simulink model "Discrete_PID_Rotate_to_Angle"  (R2020a)
settings: Solver=VariableStepAuto  StartTime=0.0  StopTime=10.0  RelTol=1e-3
libraries: simulink x2
settings Model: Creator=tieub  LastModifiedBy=tieub

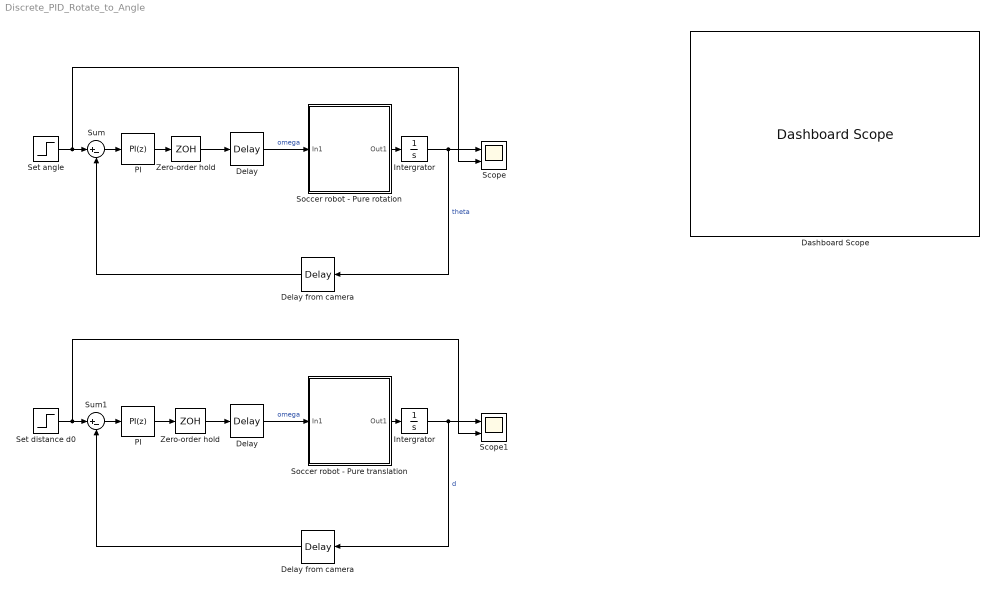
== system Discrete_PID_Rotate_to_Angle ==
  Dashboard Scope : DashboardScope
  Delay : TransportDelay  DelayTime=0.1
  "Delay " : TransportDelay  DelayTime=0.05
  Delay from camera : TransportDelay  DelayTime=0.1
  "Delay from camera " : TransportDelay  DelayTime=0.05
  Intergrator : Integrator  WrapState=on
  "Intergrator " : Integrator
  PI : simulink/Continuous/PID Controller  Controller=PI  Form=Parallel  TimeDomain=Discrete-time  UseExternalTs=off  SampleTime=0.05  IntegratorMethod=Forward Euler  FilterMethod=Forward Euler  ControllerParametersSource=internal  P=8.02568576328399  I=0.0767163752752602  D=1.24615307073805  UseFilter=off  N=69.3048635584527  TunerSelectOption=Transfer Function Based (PID Tuner App)  InitialConditionSource=internal  InitialConditionForIntegrator=0  InitialConditionForFilter=0  DifferentiatorICPrevScaledInput=0  ExternalReset=none  TrackingMode=off  Kt=1  LimitOutput=on  UpperSaturationLimit=150  LowerSaturationLimit=-150  LinearizeAsGain=off  AntiWindupMode=none  Kb=1  POutMin=[]  POutMax=[]  IOutMin=[]  IOutMax=[]  DOutMin=[]  DOutMax=[]  NOutMin=[]  NOutMax=[]  SumOutMin=[]  SumOutMax=[]  SaturationOutMin=[]  SaturationOutMax=[]  PParamMin=[]  PParamMax=[]  IParamMin=[]  IParamMax=[]  DParamMin=[]  DParamMax=[]  NParamMin=[]  NParamMax=[]  KbParamMin=[]  KbParamMax=[]  KtParamMin=[]  KtParamMax=[]  KbOutMin=[]  KbOutMax=[]  KtOutMin=[]  KtOutMax=[]  IntegratorOutMin=[]  IntegratorOutMax=[]  FilterOutMin=[]  FilterOutMax=[]  SumI1OutMin=[]  SumI1OutMax=[]  SumI2OutMin=[]  SumI2OutMax=[]  SumI3OutMin=[]  SumI3OutMax=[]  SumI4OutMin=[]  SumI4OutMax=[]  SumDOutMin=[]  SumDOutMax=[]  DifferentiatorOutMin=[]  DifferentiatorOutMax=[]  FilterDiffOutCoefMin=[]  FilterDiffOutCoefMax=[]  ReciprocalOutMin=[]  ReciprocalOutMax=[]  SumDenOutMin=[]  SumDenOutMax=[]  SumNumOutMin=[]  SumNumOutMax=[]  DivideOutMin=[]  DivideOutMax=[]  UdiffTsProdOutMin=[]  UdiffTsProdOutMax=[]  NTsProdOutMin=[]  NTsProdOutMax=[]  UintegralTsProdOutMin=[]  UintegralTsProdOutMax=[]  UngainTsProdOutMin=[]  UngainTsProdOutMax=[]  IntegratorContinuousStateAttributes=''  IntegratorStateMustResolveToSignalObject=off  IntegratorRTWStateStorageClass=Auto  FilterContinuousStateAttributes=''  FilterStateMustResolveToSignalObject=off  FilterRTWStateStorageClass=Auto  ParallelPVariant=InternalParameters  IdealPVariant=Disabled  IVariant=InternalParameters  DVariant=Disabled  IntegratorVariant=Discrete  SatVariant=Enabled  AWVariant=Passthrough  PCopyVariant=Disabled  TRVariant=Disabled  FdbkBlocksVariant=Forward  IdealPFdbkVariant=Disabled  SatFdbkVariant=Disabled  DerivativeFilterVariant=Disabled  NVariant=Disabled  NCopyVariant=Disabled_SignalSpec  FilterICVariant=Disabled  IntegratorICVariant=InternalICs  ExternalResetVariant=Disabled  TRSumVariant=Passthrough  SumFdbkVariant=Disabled  SumVariant=Sum_PI  TsampFilterVariant=InternalTs  TsampNgainVariant=Passthrough  TsampIntegralVariant=Passthrough
  "PI " : simulink/Continuous/PID Controller  Controller=PI  Form=Parallel  TimeDomain=Discrete-time  UseExternalTs=off  SampleTime=0.05  IntegratorMethod=Forward Euler  FilterMethod=Forward Euler  ControllerParametersSource=internal  P=160.51371526622  I=1.53432750551073  D=1.24615307073805  UseFilter=off  N=69.3048635584527  TunerSelectOption=Transfer Function Based (PID Tuner App)  InitialConditionSource=internal  InitialConditionForIntegrator=0  InitialConditionForFilter=0  DifferentiatorICPrevScaledInput=0  ExternalReset=none  TrackingMode=off  Kt=1  LimitOutput=on  UpperSaturationLimit=150  LowerSaturationLimit=-150  LinearizeAsGain=off  AntiWindupMode=none  Kb=1  POutMin=[]  POutMax=[]  IOutMin=[]  IOutMax=[]  DOutMin=[]  DOutMax=[]  NOutMin=[]  NOutMax=[]  SumOutMin=[]  SumOutMax=[]  SaturationOutMin=[]  SaturationOutMax=[]  PParamMin=[]  PParamMax=[]  IParamMin=[]  IParamMax=[]  DParamMin=[]  DParamMax=[]  NParamMin=[]  NParamMax=[]  KbParamMin=[]  KbParamMax=[]  KtParamMin=[]  KtParamMax=[]  KbOutMin=[]  KbOutMax=[]  KtOutMin=[]  KtOutMax=[]  IntegratorOutMin=[]  IntegratorOutMax=[]  FilterOutMin=[]  FilterOutMax=[]  SumI1OutMin=[]  SumI1OutMax=[]  SumI2OutMin=[]  SumI2OutMax=[]  SumI3OutMin=[]  SumI3OutMax=[]  SumI4OutMin=[]  SumI4OutMax=[]  SumDOutMin=[]  SumDOutMax=[]  DifferentiatorOutMin=[]  DifferentiatorOutMax=[]  FilterDiffOutCoefMin=[]  FilterDiffOutCoefMax=[]  ReciprocalOutMin=[]  ReciprocalOutMax=[]  SumDenOutMin=[]  SumDenOutMax=[]  SumNumOutMin=[]  SumNumOutMax=[]  DivideOutMin=[]  DivideOutMax=[]  UdiffTsProdOutMin=[]  UdiffTsProdOutMax=[]  NTsProdOutMin=[]  NTsProdOutMax=[]  UintegralTsProdOutMin=[]  UintegralTsProdOutMax=[]  UngainTsProdOutMin=[]  UngainTsProdOutMax=[]  IntegratorContinuousStateAttributes=''  IntegratorStateMustResolveToSignalObject=off  IntegratorRTWStateStorageClass=Auto  FilterContinuousStateAttributes=''  FilterStateMustResolveToSignalObject=off  FilterRTWStateStorageClass=Auto  ParallelPVariant=InternalParameters  IdealPVariant=Disabled  IVariant=InternalParameters  DVariant=Disabled  IntegratorVariant=Discrete  SatVariant=Enabled  AWVariant=Passthrough  PCopyVariant=Disabled  TRVariant=Disabled  FdbkBlocksVariant=Forward  IdealPFdbkVariant=Disabled  SatFdbkVariant=Disabled  DerivativeFilterVariant=Disabled  NVariant=Disabled  NCopyVariant=Disabled_SignalSpec  FilterICVariant=Disabled  IntegratorICVariant=InternalICs  ExternalResetVariant=Disabled  TRSumVariant=Passthrough  SumFdbkVariant=Disabled  SumVariant=Sum_PI  TsampFilterVariant=InternalTs  TsampNgainVariant=Passthrough  TsampIntegralVariant=Passthrough
  Scope : Scope  NumInputPorts=2
  Scope1 : Scope  NumInputPorts=2
  Set angle : Step  Time=0  SampleTime=0
  Set distance d0 : Step  Time=0  SampleTime=0
  Soccer robot - Pure rotation : Subsystem
      mask Display: image('G:\Shared drives\Study Group\THESISISISISISISISISISISISIS\Gallery\robot.jpg'); % Use "Edit Image" on toolstrip to change.
  Soccer robot - Pure translation : Subsystem
      mask Display: image('G:\Shared drives\Study Group\THESISISISISISISISISISISISIS\Gallery\robot.jpg'); % Use "Edit Image" on toolstrip to change.
  Sum : Sum  Inputs=|+-
  Sum1 : Sum  Inputs=|+-
  Zero-order hold : ZeroOrderHold  SampleTime=0.05
  "Zero-order hold " : ZeroOrderHold  SampleTime=0.05
  wires:
  Sum/1 -> PI/1
  Set angle/1 -> Scope/2, Sum/1
  PI/1 -> Zero-order hold/1
  Delay from camera/1 -> Sum/2
  Delay/1 -> Soccer robot - Pure rotation/1(In1)  "omega"
  Soccer robot - Pure rotation/1(Out1) -> Intergrator/1
  Intergrator/1 -> Delay from camera/1, Scope/1  "theta"
  Zero-order hold/1 -> Delay/1
  "Zero-order hold "/1 -> "Delay "/1
  Set distance d0/1 -> Scope1/2, Sum1/1
  Soccer robot - Pure translation/1(Out1) -> "Intergrator "/1
  "Delay "/1 -> Soccer robot - Pure translation/1(In1)  "omega"
  "Intergrator "/1 -> "Delay from camera "/1, Scope1/1  "d"
  "Delay from camera "/1 -> Sum1/2
  "PI "/1 -> "Zero-order hold "/1
  Sum1/1 -> "PI "/1

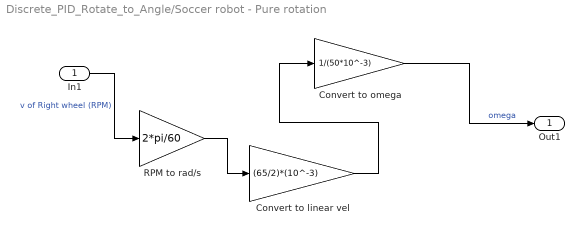
== system Discrete_PID_Rotate_to_Angle/Soccer robot - Pure rotation ==
  In1 : Inport
  Convert to linear vel : Gain  Gain=(65/2)*(10^-3)
  Convert to omega : Gain  Gain=1/(50*10^-3)
  RPM to rad/s : Gain  Gain=2*pi/60
  Out1 : Outport
  wires:
  In1/1 -> RPM to rad/s/1  "v of Right wheel (RPM)"
  RPM to rad/s/1 -> Convert to linear vel/1
  Convert to linear vel/1 -> Convert to omega/1
  Convert to omega/1 -> Out1/1  "omega"

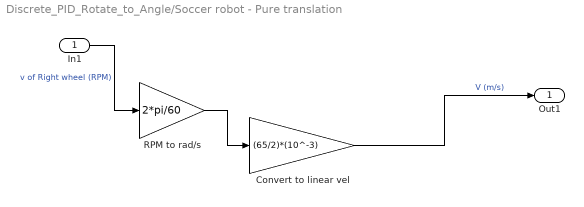
== system Discrete_PID_Rotate_to_Angle/Soccer robot - Pure translation ==
  In1 : Inport
  Convert to linear vel : Gain  Gain=(65/2)*(10^-3)
  RPM to rad/s : Gain  Gain=2*pi/60
  Out1 : Outport
  wires:
  In1/1 -> RPM to rad/s/1  "v of Right wheel (RPM)"
  RPM to rad/s/1 -> Convert to linear vel/1
  Convert to linear vel/1 -> Out1/1  "V (m/s)"
